simulink model "LinLongNormal_Aquila_ClawsGainSchedule_Discrete"  (R2017a)
settings: Solver=VariableStepAuto  StartTime=0.0  StopTime=50  RelTol=1e-3  EnableMultiTasking=on
PreLoadFcn:
  | AquilaDiscreteClawsParameters_GS
  | AquilaDiscreteModelParameters
model workspace: external: MAT-File (data not in the file)
undefined symbols (not defined in the file): AP_AltLoop_AltCmdLPFDenTau, AP_AltLoop_Kd0, AP_AltLoop_Ki0, AP_AltLoop_Ki_WindupMaxLim, AP_AltLoop_Ki_WindupMinLim, AP_AltLoop_Kp0, AP_ClimbRate_LPFDenTau, AP_ClimbRateLoop_ClimbRateCmdLPFDenTau, AP_ClimbRateLoop_Ki0, AP_ClimbRateLoop_Kp0, AP_ClimbRateLoop_LLFiltDenCoe0, AP_ClimbRateLoop_LLFiltNumCoe0, AP_ClimbRateLoop_MaxPitchCmdrad, AP_ClimbRateLoop_MinPitchCmdrad, AP_GndTrkLoop_CmdLPFDenTau, AP_GndTrkLoop_Kd0, AP_GndTrkLoop_Kp0, AP_GndTrkLoop_phiCmdMaxLimDeg, AP_GndTrkLoop_phiCmdMinLimDeg, AP_GndTrkLoop_phiRateCmdMaxLimDps, AP_GndTrkLoop_phiRateCmdMinLimDps, AP_PitchLoop_DerivLPFDenTau, AP_PitchLoop_Kd, AP_PitchLoop_Kff, AP_PitchLoop_Ki0, AP_PitchLoop_Kp0, AP_PitchLoop_Kq0, AP_PitchLoop_Notch1BWfactor, AP_PitchLoop_Notch1CosFreqNorm, AP_PitchLoop_qFdbkLFLLFiltDenCoe0, AP_PitchLoop_qFdbkLFLLFiltNumCoe0, AP_PitchLoop_qFdbkLLFiltDenCoe0, AP_PitchLoop_qFdbkLLFiltNumCoe0, AP_PitchLoop_thetaCmdLPFDenTau, AP_PitchLoop_wn_ElvRollOff, AP_PitchLoop_zeta_ElvRollOff, AP_PwrLoop_ClimbRateCmdLPFDenTau, AP_PwrLoop_Ki0, AP_PwrLoop_Kp0, AP_PwrLoop_Kvadv0, AP_PwrLoop_LLFiltDenCoe0, AP_PwrLoop_LLFiltNumCoe0, AP_PwrLoop_MaxThrCmdNorm, AP_PwrLoop_MinThrCmdNorm, AP_PwrLoop_wn_ThrRollOff, AP_PwrLoop_zeta_ThrRollOff, AP_RollLoop_ailCmdMaxLim, AP_RollLoop_ailCmdMinLim, AP_RollLoop_AilWindupMaxLim, AP_RollLoop_AilWindupMinLim, AP_RollLoop_Ki0, AP_RollLoop_Kp0, AP_RollLoop_KrollrateAdv0, AP_RollLoop_Notch1BWfactor, AP_RollLoop_Notch1CosFreqNorm, AP_RollLoop_pFdbkLFLLFiltDenCoe0, AP_RollLoop_pFdbkLFLLFiltNumCoe0, AP_RollLoop_pFdbkLLFiltDenCoe0, AP_RollLoop_pFdbkLLFiltNumCoe0, AP_RollLoop_phiErrLPFDenTau ... (+41)
libraries: discretizing x16, aerolibconvert2 x12, simulink x8
(part 1 of 2)
settings Model: Creator=The MathWorks, Inc.  LastModifiedBy=hbolandhemmat
settings DataIOCC: LimitDataPoints=on
settings OptimizationCC: LifeSpan=inf
settings DebuggingCC: AllowSymbolicDim=off  SFUnexpectedBacktrackingDiag=warning  SFNoUnconditionalDefaultTransitionDiag=warning  SFExecutionAtInitializationDiag=none
settings ModelReferenceCC: PropagateSignalLabelsOutOfModel=off
settings GRTTargetCC: TargetLangStandard=C89/C90 (ANSI)
settings ConfigComp: CovMetricSettings=dw  CovHtmlReporting=on  CovSaveCumulativeToWorkspaceVar=on  CovSaveSingleToWorkspaceVar=on  CovExternalEMLEnable=off

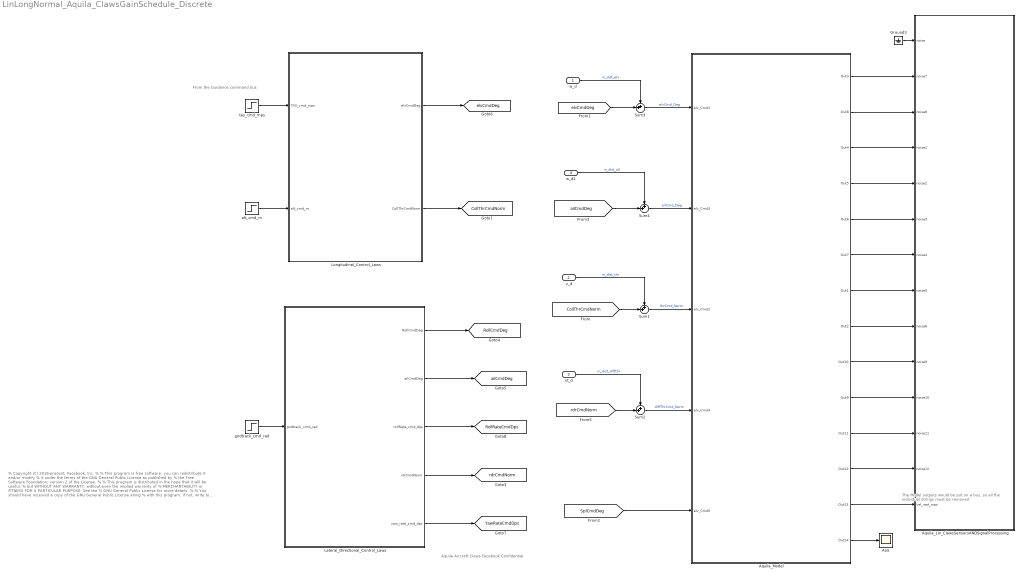
== system LinLongNormal_Aquila_ClawsGainSchedule_Discrete ==
  note: From the Guidance command bus
  note: Aquila Aircraft Claws
      | Facebook Confidential
  note: The Model outputs would be put on a bus, so all
      | the individual strings must be removed
  note: % Copyright (C) 2018-present, Facebook, Inc.
      | %
      | % This program is free software; you can redistribute it and/or modify
      | % it under the terms of the GNU General Public License as published by
      | % the Free Software Foundation; version 2 of the License.
      | %
      | % This program is distributed in the hope that it will be useful,
      | % but WITHOUT ANY WARRANTY; without even the implied warranty of
      | % MERCHANTABILITY or FITNESS FOR A PARTICULAR PURPOSE. See the
      | % GNU General Public License for more details.
      | %
      | % You should have received a copy of the GNU General Public License along
      | % with this program; if not, write to the Free Software Foundation, Inc.,
      | % 51 Franklin Street, Fifth Floor, Boston, MA 02110-1301 USA.
  w_d : Inport
  v_d : Inport  Port=2
  nt_d : Inport  Port=3
  w_d1 : Inport  Port=4
  AoS : Scope
  Aquila_Lin_ClawsSensorsANDSignalProcessing : Subsystem
  Aquila_Model : Subsystem
  Ground3 : Ground
  Lateral_Directional_Control_Laws : Subsystem
  Longitudinal_Control_Laws : Subsystem
  Sum{1..4} (4 alike) : Sum  Inputs=++|
  alt_cmd_m : Step  After=0  SampleTime=0
  gndtrack_cmd_rad : Step  SampleTime=0
  tas_cmd_mps : Step  After=0  SampleTime=0
  tag scope: CollThrCmdNorm=global, RollCmdDeg=global, RollRateCmdDps=global, YawRateCmdDps=global, ailCmdDeg=global, elvCmdDeg=global, rdrCmdNorm=global
  wires:
  alt_cmd_m/1 -> Longitudinal_Control_Laws/2(alt_cmd_m)
  Longitudinal_Control_Laws/1(elvCmdDeg) -> [elvCmdDeg]
  Longitudinal_Control_Laws/2(CollThrCmdNorm) -> [CollThrCmdNorm]
  w_d/1 -> Sum3/1  "in_dist_elv"
  Sum3/1 -> Aquila_Model/1(elv_Cmd1)  "elvCmd_Deg"
  Ground3/1 -> Aquila_Lin_ClawsSensorsANDSignalProcessing/1(noise)
  Aquila_Model/4(Out5) -> Aquila_Lin_ClawsSensorsANDSignalProcessing/5(noise2)
  Aquila_Model/3(Out4) -> Aquila_Lin_ClawsSensorsANDSignalProcessing/4(noise1)
  Aquila_Model/6(Out7) -> Aquila_Lin_ClawsSensorsANDSignalProcessing/7(noise4)
  Aquila_Model/1(Out3) -> Aquila_Lin_ClawsSensorsANDSignalProcessing/2(noise7)
  Aquila_Model/7(Out1) -> Aquila_Lin_ClawsSensorsANDSignalProcessing/8(noise5)
  Aquila_Model/8(Out2) -> Aquila_Lin_ClawsSensorsANDSignalProcessing/9(noise6)
  Aquila_Model/2(Out8) -> Aquila_Lin_ClawsSensorsANDSignalProcessing/3(noise8)
  v_d/1 -> Sum1/1  "in_dist_thr"
  Sum1/1 -> Aquila_Model/3(elv_Cmd2)  "thrCmd_Norm"
  Aquila_Model/5(Out6) -> Aquila_Lin_ClawsSensorsANDSignalProcessing/6(noise3)
  tas_cmd_mps/1 -> Longitudinal_Control_Laws/1(TAS_cmd_mps)
  [CollThrCmdNorm] -> Sum1/2
  [elvCmdDeg] -> Sum3/2
  Aquila_Model/9(Out10) -> Aquila_Lin_ClawsSensorsANDSignalProcessing/10(noise9)
  Aquila_Model/10(Out9) -> Aquila_Lin_ClawsSensorsANDSignalProcessing/11(noise10)
  Aquila_Model/11(Out11) -> Aquila_Lin_ClawsSensorsANDSignalProcessing/12(noise11)
  Aquila_Model/12(Out12) -> Aquila_Lin_ClawsSensorsANDSignalProcessing/13(noise12)
  Aquila_Model/13(Out13) -> Aquila_Lin_ClawsSensorsANDSignalProcessing/14(vel_ned_mps)
  Sum2/1 -> Aquila_Model/4(elv_Cmd4)  "diffThrCmd_Norm"
  [rdrCmdNorm] -> Sum2/2
  nt_d/1 -> Sum2/1  "in_dist_diffthr"
  Aquila_Model/14(Out14) -> AoS/1
  w_d1/1 -> Sum4/1  "in_dist_ail"
  [ailCmdDeg] -> Sum4/2
  Sum4/1 -> Aquila_Model/2(elv_Cmd3)  "ailCmd_Deg"
  [SplCmdDeg] -> Aquila_Model/5(elv_Cmd5)
  gndtrack_cmd_rad/1 -> Lateral_Directional_Control_Laws/1(gndtrack_cmd_rad)
  Lateral_Directional_Control_Laws/2(ailCmdDeg) -> [ailCmdDeg]
  Lateral_Directional_Control_Laws/1(RollCmdDeg) -> [RollCmdDeg]
  Lateral_Directional_Control_Laws/4(rdrCmdNorm) -> [rdrCmdNorm]
  Lateral_Directional_Control_Laws/5(yaw_rate_cmd_dps) -> [YawRateCmdDps]
  Lateral_Directional_Control_Laws/3(rollRate_cmd_dps) -> [RollRateCmdDps]

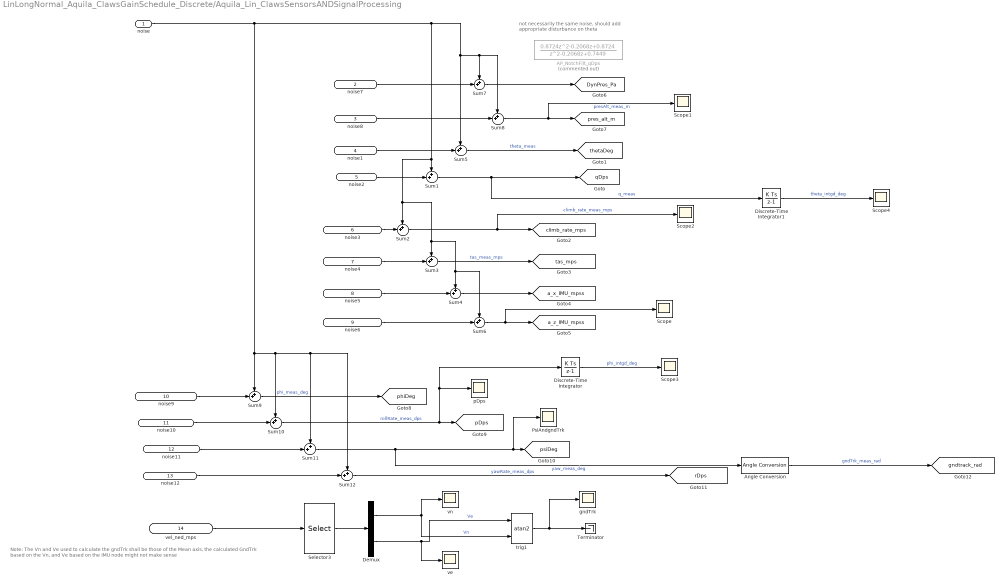
== system LinLongNormal_Aquila_ClawsGainSchedule_Discrete/Aquila_Lin_ClawsSensorsANDSignalProcessing ==
  note: Note: The Vn and Ve used to calculate the gndTrk shall be those of the Mean axis, the
      | calculated GndTrk based on the Vn, and Ve based on the IMU node might not make sense
  note: not necessarily the same noise,
      | should add appropriate disturbance on theta
  noise : Inport
  noise7 : Inport  Port=2
  noise8 : Inport  Port=3
  noise1 : Inport  Port=4
  noise2 : Inport  Port=5
  noise3 : Inport  Port=6
  noise4 : Inport  Port=7
  noise5 : Inport  Port=8
  noise6 : Inport  Port=9
  noise9 : Inport  Port=10
  noise10 : Inport  Port=11
  noise11 : Inport  Port=12
  noise12 : Inport  Port=13
  vel_ned_mps : Inport  Port=14
  AP_NotchFilt_qDps : DiscreteTransferFcn  Commented=on  Numerator=[0.8724 -0.2068 0.8724]  Denominator=[1 -0.2068 0.7449]  SampleTime=Ts
  Angle Conversion : aerolibconvert2/Angle Conversion  IU=deg  OU=rad
  Demux : Demux  Outputs=2
  Discrete-Time Integrator : DiscreteIntegrator  gainval=1  InitialConditionSetting=State (most efficient)  SampleTime=-1  ICPrevOutput=DiscIntNeverNeededParam  ICPrevScaledInput=DiscIntNeverNeededParam
  Discrete-Time Integrator1 : DiscreteIntegrator  gainval=1  InitialConditionSetting=State (most efficient)  SampleTime=-1  ICPrevOutput=DiscIntNeverNeededParam  ICPrevScaledInput=DiscIntNeverNeededParam
  PsiAndgndTrk : Scope
  Scope{,1..4} (5 alike) : Scope
  Selector3 : Selector  InputPortWidth=3  IndexOptions=Index vector (dialog)  Indices=1:2  OutputSizes=1
  Sum{1..12} (12 alike) : Sum  Inputs=++|
  Terminator : Terminator
  gndTrk : Scope
  pDps : Scope
  trig1 : Trigonometry  Operator=atan2
  ve : Scope
  vn : Scope
  tag scope: DynPres_Pa=global, a_x_IMU_mpss=global, a_z_IMU_mpss=global, climb_rate_mps=global, gndtrack_rad=global, pDps=global, phiDeg=global, pres_alt_m=global, psiDeg=global, qDps=global, rDps=global, tas_mps=global, thetaDeg=global
  wires:
  noise1/1 -> Sum5/2
  noise2/1 -> Sum1/2
  Sum5/1 -> [thetaDeg]  "theta_meas"
  Sum1/1 -> Discrete-Time Integrator1/1, [qDps]  "q_meas"
  noise3/1 -> Sum2/2
  Sum2/1 -> Scope2/1, [climb_rate_mps]  "climb_rate_meas_mps"
  noise4/1 -> Sum3/2
  Sum3/1 -> [tas_mps]  "tas_meas_mps"
  noise5/1 -> Sum4/2
  Sum4/1 -> [a_x_IMU_mpss]
  noise6/1 -> Sum6/2
  Sum6/1 -> Scope/1, [a_z_IMU_mpss]
  noise7/1 -> Sum7/2
  Sum7/1 -> [DynPres_Pa]
  noise8/1 -> Sum8/2
  Sum8/1 -> Scope1/1, [pres_alt_m]  "presAlt_meas_m"
  noise9/1 -> Sum9/2
  noise/1 -> Sum12/1, Sum11/1, Sum10/1, Sum9/1, Sum5/1, Sum8/1, Sum7/1, Sum6/1, Sum4/1, Sum3/1, Sum2/1, Sum1/1
  noise10/1 -> Sum10/2
  noise12/1 -> Sum12/2
  noise11/1 -> Sum11/2
  Sum9/1 -> [phiDeg]  "phi_meas_deg"
  Sum10/1 -> Discrete-Time Integrator/1, pDps/1, [pDps]  "rollRate_meas_dps"
  Sum11/1 -> PsiAndgndTrk/1, [psiDeg], Angle Conversion/1  "yaw_meas_deg"
  Sum12/1 -> [rDps]  "yawRate_meas_dps"
  Selector3/1 -> Demux/1
  Demux/2 -> trig1/1, ve/1  "Ve"
  Demux/1 -> vn/1, trig1/2  "Vn"
  vel_ned_mps/1 -> Selector3/1
  trig1/1 -> Terminator/1, gndTrk/1
  Angle Conversion/1 -> [gndtrack_rad]  "gndTrk_meas_rad"
  Discrete-Time Integrator/1 -> Scope3/1  "phi_intgd_deg"
  Discrete-Time Integrator1/1 -> Scope4/1  "theta_intgd_deg"

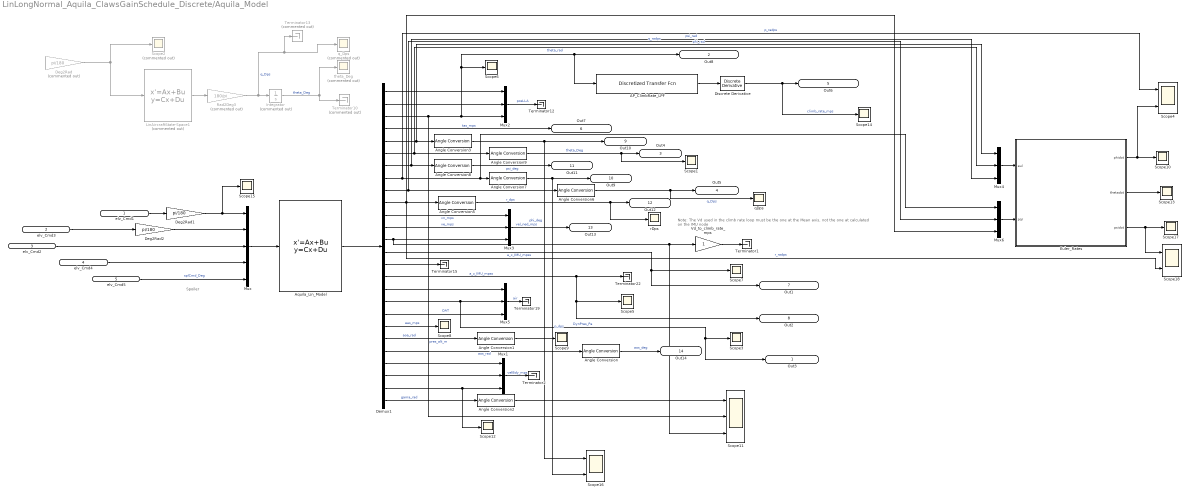
== system LinLongNormal_Aquila_ClawsGainSchedule_Discrete/Aquila_Model ==
  note: Spoiler
  note: Note: The Vd used in the climb rate loop must be the one at the Mean axis,
      | not the one at calculated on the IMU node
  elv_Cmd1 : Inport
  elv_Cmd3 : Inport  Port=2
  elv_Cmd2 : Inport  Port=3
  elv_Cmd4 : Inport  Port=4
  elv_Cmd5 : Inport  Port=5
  AP_ClimbRate_LPF : discretizing/Discretized Transfer Fcn  Numerator=[1]  Denominator=[AP_ClimbRate_LPFDenTau 1]  AbsTol=auto  SampleTime=Ts  method=zoh  Wc=1
  Angle Conversion{,1..3,5..9} (9 alike) : aerolibconvert2/Angle Conversion  IU=rad  OU=deg
  Aquila_Lin_Model : StateSpace  A=LIN_AC_S_A  B=LIN_AC_S_B  C=LIN_AC_S_C  D=LIN_AC_S_D  X0=0
  Deg2Rad : Gain  Commented=on  Gain=pi/180
  Deg2Rad1 : Gain  Gain=pi/180
  Deg2Rad2 : Gain  Gain=pi/180
  Demux1 : Demux  Outputs=26
  Discrete Derivative : simulink/Discrete/Discrete Derivative  gainval=1.0  ICPrevScaledInput=0.0  OutMin=[]  OutMax=[]  OutDataType=fixdt(1, 16)  OutScaling=2^-10  DoSatur=off
  Euler_Rates : Subsystem
  Integrator : Integrator  Commented=on
  LinAircraftState-Space1 : StateSpace  Commented=on  A=LIN_AC_S_A  B=LIN_AC_S_B  C=LIN_AC_S_C  D=LIN_AC_S_D  X0=0
  Mux : Mux  Inputs=5
  Mux{1..6} (6 alike) : Mux  Inputs=3
  Rad2Deg3 : Gain  Commented=on  Gain=180/pi
  Scope{1,3,5..10,12..15,17} (13 alike) : Scope
  Scope11 : Scope  NumInputPorts=3
  Scope16 : Scope  NumInputPorts=2
  Scope18 : Scope  NumInputPorts=2
  Scope2 : Scope  Commented=on
  Scope4 : Scope  NumInputPorts=2
  Terminator{1..2,12,15,19,22} (6 alike) : Terminator
  Terminator10 : Terminator  Commented=on
  Terminator13 : Terminator  Commented=on
  Vd_to_climb_rate_mps : Gain
  qDps : Scope
  q_Dps : Scope  Commented=on
  rDps : Scope
  theta_Deg : Scope  Commented=on
  Out3 : Outport
  Out8 : Outport  Port=2
  Out4 : Outport  Port=3
  Out5 : Outport  Port=4
  Out6 : Outport  Port=5
  Out7 : Outport  Port=6
  Out1 : Outport  Port=7
  Out2 : Outport  Port=8
  Out10 : Outport  Port=9
  Out9 : Outport  Port=10
  Out11 : Outport  Port=11
  Out12 : Outport  Port=12
  Out13 : Outport  Port=13
  Out14 : Outport  Port=14
  wires:
  LinAircraftState-Space1/1 -> Rad2Deg3/1
  Deg2Rad/1 -> LinAircraftState-Space1/1, Scope2/1
  Integrator/1 -> Terminator10/1, theta_Deg/1  "theta_Deg"
  Rad2Deg3/1 -> q_Dps/1, Terminator13/1, Integrator/1  "q_Dps"
  elv_Cmd5/1 -> Mux/5  "splCmd_Deg"
  Mux/1 -> Aquila_Lin_Model/1
  Deg2Rad1/1 -> Scope15/1, Mux/1
  elv_Cmd1/1 -> Deg2Rad1/1
  Demux1/8 -> Scope4/1, Mux6/1, Angle Conversion7/1  "p_radps"
  Demux1/15 -> Terminator15/1
  Demux1/3 -> Scope6/1, AP_ClimbRate_LPF/1, Out8/1, Mux2/3, Scope11/2  "pres_alt_m"
  Mux2/1 -> Terminator12/1  "posLLA"
  Demux1/2 -> Mux2/2
  Demux1/18 -> Out3/1, Scope3/1, Mux5/2  "DynPres_Pa"
  Demux1/17 -> Mux5/1
  Demux1/1 -> Mux2/1
  Demux1/19 -> Mux5/3  "OAT"
  Mux5/1 -> Terminator19/1  "air"
  Demux1/5 -> Mux4/1, Angle Conversion3/1  "phi_rad"
  Demux1/14 -> Out1/1, Scope7/1  "a_x_IMU_mpss"
  Demux1/16 -> Out2/1, Scope5/1, Terminator22/1  "a_z_IMU_mpss"
  Demux1/7 -> Mux4/3, Angle Conversion8/1  "psi_rad"
  Demux1/6 -> Mux4/2, Angle Conversion9/1  "theta_rad"
  Angle Conversion9/1 -> Scope1/1, Out4/1  "theta_Deg"
  Demux1/9 -> Mux6/2, Angle Conversion6/1  "q_radps"
  Angle Conversion6/1 -> qDps/1, Out5/1  "q_Dps"
  Aquila_Lin_Model/1 -> Demux1/1
  Demux1/4 -> Out7/1  "tas_mps"
  Vd_to_climb_rate_mps/1 -> Terminator1/1
  Demux1/20 -> Scope8/1  "eas_mps"
  Demux1/21 -> Angle Conversion1/1  "aoa_rad"
  Demux1/22 -> Angle Conversion/1  "aos_rad"
  Demux1/23 -> Mux1/1
  Demux1/24 -> Mux1/2
  Demux1/26 -> Angle Conversion2/1  "gama_rad"
  Angle Conversion/1 -> Out14/1  "aos_deg"
  Angle Conversion1/1 -> Scope9/1
  Angle Conversion2/1 -> Scope11/1
  elv_Cmd4/1 -> Mux/4
  AP_ClimbRate_LPF/1 -> Discrete Derivative/1
  Discrete Derivative/1 -> Scope14/1, Out6/1  "climb_rate_mps"
  Demux1/10 -> Scope18/2, Mux6/3, Angle Conversion5/1  "r_radps"
  Angle Conversion5/1 -> rDps/1, Out12/1  "r_dps"
  Angle Conversion7/1 -> Scope16/2, Out9/1  "p_dps"
  Angle Conversion3/1 -> Scope16/1, Out10/1  "phi_deg"
  Angle Conversion8/1 -> Out11/1  "psi_deg"
  elv_Cmd2/1 -> Mux/3
  elv_Cmd3/1 -> Deg2Rad2/1
  Mux1/1 -> Terminator2/1  "velBdy_mps"
  Demux1/25 -> Scope12/1, Mux1/3
  Demux1/11 -> Mux3/1  "vn_mps"
  Demux1/12 -> Mux3/2  "ve_mps"
  Demux1/13 -> Scope11/3, Vd_to_climb_rate_mps/1, Mux3/3
  Mux3/1 -> Out13/1  "vel_ned_mps"
  Mux4/1 -> Euler_Rates/1(eul)
  Mux6/1 -> Euler_Rates/2(pqr)
  Euler_Rates/1(phidot) -> Scope4/2, Scope10/1
  Euler_Rates/2(thetadot) -> Scope13/1
  Euler_Rates/3(psidot) -> Scope18/1, Scope17/1
  Deg2Rad2/1 -> Mux/2

== system LinLongNormal_Aquila_ClawsGainSchedule_Discrete/Lateral_Directional_Control_Laws ==
  note: Aquila Aircraft Claws
      | Facebook Confidential
  gndtrack_cmd_rad : Inport
  GndTrkLoop : Subsystem
  RollLoop : Subsystem
  YawLoop : Subsystem
  RollCmdDeg : Outport
  ailCmdDeg : Outport  Port=2
  rollRate_cmd_dps : Outport  Port=3
  rdrCmdNorm : Outport  Port=4
  yaw_rate_cmd_dps : Outport  Port=5
  wires:
  gndtrack_cmd_rad/1 -> GndTrkLoop/1(alt_cmd_m)
  RollLoop/1(ail_cmd_RollRateLoop_deg) -> ailCmdDeg/1
  YawLoop/1(Rdr_cmd_YawRateLoop_norm) -> rdrCmdNorm/1
  YawLoop/2(yaw_rate_cmd_dps) -> yaw_rate_cmd_dps/1
  GndTrkLoop/1(Phi_cmd_deg) -> RollCmdDeg/1, RollLoop/1(phi_cmd_deg)
  RollLoop/3(phi_err_filt) -> YawLoop/1(alt_cmd_m)
  RollLoop/2(PhiRateCmd_Dps) -> rollRate_cmd_dps/1
  GndTrkLoop/2(PhiRate_cmd_dps) -> RollLoop/2(phiRateCmd_Dps)

== system LinLongNormal_Aquila_ClawsGainSchedule_Discrete/Longitudinal_Control_Laws ==
  note: The ClimbRate loop might be replaced by the Nz loop
      | in the future depending on the overall loop performance
      | and availability of the Nz signal in terms of SNR
  note: Aquila Aircraft Longitudinal Claws
      | Facebook Confidential
  TAS_cmd_mps : Inport
  alt_cmd_m : Inport  Port=2
  AltitudeLoop : Subsystem
  ClimbRateLoop : Subsystem
  PitchLoop : Subsystem
  PwrLoop : Subsystem
  SpeedLoop : Subsystem
  elvCmdDeg : Outport
  CollThrCmdNorm : Outport  Port=2
  wires:
  PitchLoop/1(elv_Cmd_PitchLoop) -> elvCmdDeg/1  "elvCmdDeg_PitchLoop"
  PwrLoop/1(CollThr_Cmd_PwrLoop) -> CollThrCmdNorm/1
  alt_cmd_m/1 -> AltitudeLoop/1(alt_cmd_m)
  [climb_rate_mps] -> PwrLoop/2(climb_rate_mps)
  [climb_rate_mps] -> ClimbRateLoop/3(climb_rate_mps)
  [pres_alt_m] -> AltitudeLoop/2(alt_m)
  SpeedLoop/1(climb_rate_cmd_spdloop) -> ClimbRateLoop/1(climb_rate_cmd_spdloop)
  ClimbRateLoop/1(theta_Cmd) -> PitchLoop/1(theta_Cmd)
  [tas_mps] -> PwrLoop/3(TAS_mps)
  AltitudeLoop/1(climb_rate_cmd_altloop_mps) -> PwrLoop/1(climb_rate_altloop_cmd_mps), ClimbRateLoop/2(climb_rate_cmd_altloop_mps)
  [climb_rate_mps] -> AltitudeLoop/3(climb_rate_mps)
  TAS_cmd_mps/1 -> SpeedLoop/1(TAS_cmd_mps)
  [tas_mps] -> SpeedLoop/2(TAS_mps)

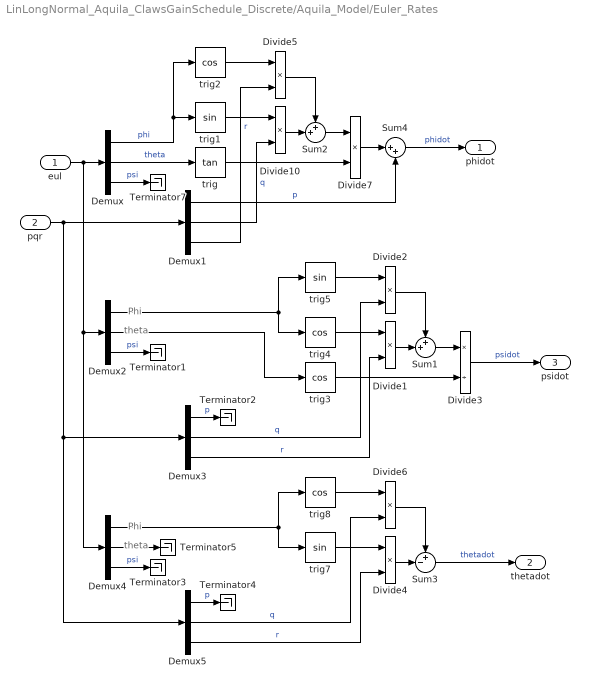
== system LinLongNormal_Aquila_ClawsGainSchedule_Discrete/Aquila_Model/Euler_Rates ==
  note: theta
  note: Phi
  note: theta
  note: Phi
  eul : Inport
  pqr : Inport  Port=2
  Demux{,1..5} (6 alike) : Demux  Outputs=3
  Divide{1..2,4..7,10} (7 alike) : Product  Inputs=**
  Divide3 : Product  Inputs=*/
  Sum1 : Sum  Inputs=++|
  Sum2 : Sum  Inputs=++|
  Sum3 : Sum  Inputs=+-|
  Sum4 : Sum  Inputs=|++
  Terminator{1..5,7} (6 alike) : Terminator
  trig : Trigonometry  Operator=tan
  trig1 : Trigonometry
  trig{2..4,8} (4 alike) : Trigonometry  Operator=cos
  trig5 : Trigonometry
  trig7 : Trigonometry
  phidot : Outport
  thetadot : Outport  Port=2
  psidot : Outport  Port=3
  wires:
  Divide5/1 -> Sum2/1
  trig2/1 -> Divide5/1
  Divide7/1 -> Sum4/1
  Demux1/1 -> Sum4/2  "p"
  trig1/1 -> Divide10/1
  Demux1/3 -> Divide5/2  "r"
  Demux1/2 -> Divide10/2  "q"
  Sum2/1 -> Divide7/1
  trig/1 -> Divide7/2
  Sum4/1 -> phidot/1  "phidot"
  Divide10/1 -> Sum2/2
  Demux/3 -> Terminator7/1  "psi"
  Divide2/1 -> Sum1/1
  trig5/1 -> Divide2/1
  trig4/1 -> Divide1/1
  Demux/1 -> trig2/1, trig1/1  "phi"
  Demux/2 -> trig/1  "theta"
  Sum1/1 -> Divide3/1
  trig3/1 -> Divide3/2
  Divide3/1 -> psidot/1  "psidot"
  Divide1/1 -> Sum1/2
  Demux3/2 -> Divide2/2  "q"
  Demux3/3 -> Divide1/2  "r"
  Demux2/1 -> trig5/1, trig4/1
  Demux2/2 -> trig3/1
  Demux2/3 -> Terminator1/1  "psi"
  Demux3/1 -> Terminator2/1  "p"
  pqr/1 -> Demux1/1, Demux3/1, Demux5/1
  Divide6/1 -> Sum3/1
  trig8/1 -> Divide6/1
  trig7/1 -> Divide4/1
  Sum3/1 -> thetadot/1  "thetadot"
  Divide4/1 -> Sum3/2
  Demux5/2 -> Divide6/2  "q"
  Demux5/3 -> Divide4/2  "r"
  eul/1 -> Demux2/1, Demux4/1, Demux/1
  Demux4/1 -> trig8/1, trig7/1
  Demux4/3 -> Terminator3/1  "psi"
  Demux5/1 -> Terminator4/1  "p"
  Demux4/2 -> Terminator5/1

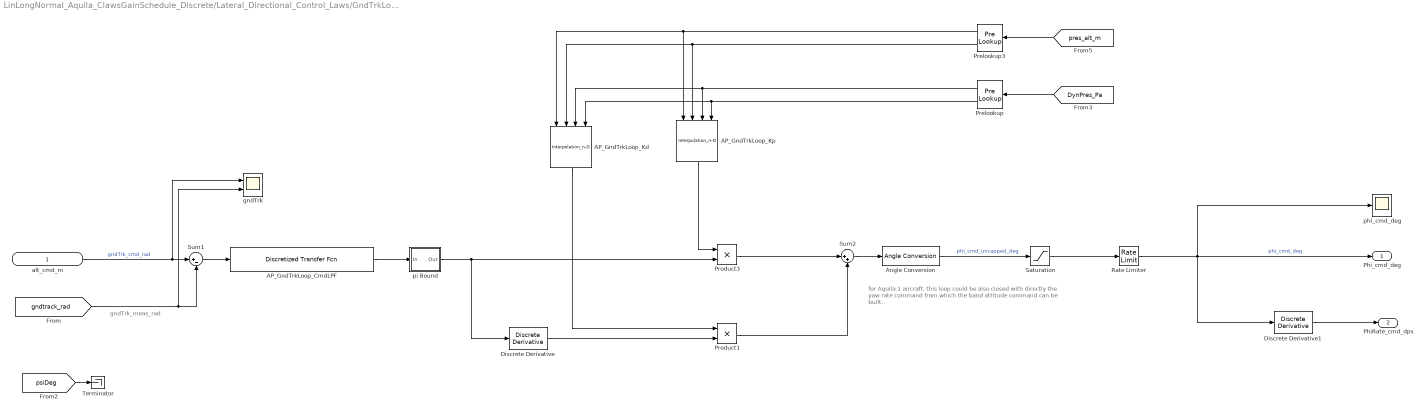
== system LinLongNormal_Aquila_ClawsGainSchedule_Discrete/Lateral_Directional_Control_Laws/GndTrkLoop ==
  note: gndTrk_meas_rad
  note: for Aquila 1 aircraft, this loop could be also closed with
      | directly the yaw rate command from which the band attitude
      | command can be built.
  alt_cmd_m : Inport
  AP_GndTrkLoop_CmdLPF : discretizing/Discretized Transfer Fcn  Numerator=[1]  Denominator=[AP_GndTrkLoop_CmdLPFDenTau 1]  AbsTol=auto  SampleTime=Ts  method=zoh  Wc=1
  AP_GndTrkLoop_Kd : Interpolation_n-D  Table=AP_GndTrkLoop_Kd0  ExtrapMethod=Clip  InternalRulePriority=Speed
  AP_GndTrkLoop_Kp : Interpolation_n-D  Table=AP_GndTrkLoop_Kp0  ExtrapMethod=Clip  InternalRulePriority=Speed
  Angle Conversion : aerolibconvert2/Angle Conversion  IU=rad  OU=deg
  Discrete Derivative : simulink/Discrete/Discrete Derivative  gainval=1.0  ICPrevScaledInput=0.0  OutMin=[]  OutMax=[]  OutDataType=fixdt(1, 16)  OutScaling=2^-10  DoSatur=off
  Discrete Derivative1 : simulink/Discrete/Discrete Derivative  gainval=1.0  ICPrevScaledInput=0.0  OutMin=[]  OutMax=[]  OutDataType=fixdt(1, 16)  OutScaling=2^-10  DoSatur=off
  Prelookup : PreLookup  BreakpointsData=45:15:150  ExtrapMethod=Linear
  Prelookup3 : PreLookup  BreakpointsData=0:1500:12000  ExtrapMethod=Linear
  Product1 : Product
  Product3 : Product
  Rate Limiter : RateLimiter  RisingSlewLimit=AP_GndTrkLoop_phiRateCmdMaxLimDps  FallingSlewLimit=AP_GndTrkLoop_phiRateCmdMinLimDps  SampleTimeMode=inherited
  Saturation : Saturate  UpperLimit=AP_GndTrkLoop_phiCmdMaxLimDeg  LowerLimit=AP_GndTrkLoop_phiCmdMinLimDeg
  Sum1 : Sum  Inputs=|+-
  Sum2 : Sum  Inputs=|++
  Terminator : Terminator
  gndTrk : Scope  NumInputPorts=2
  phi_cmd_deg : Scope
  pi Bound : Subsystem  mask(pi bound){}
      mask help: Bounds the input angle to [-pi, pi]. When -pi bound is exceeded the output wraps back to pi; when the pi bound is exceeded the output wraps back to -pi.
      mask Help:
      | Bounds the input angle to [-pi, pi]. When -pi bound is exceeded the output wraps back to pi; when the pi bound is exceeded the output wraps back to -pi.
      | <P><B>Input:</B> any angle in radians, from -Inf to Inf;</P>
      | <P><B>Output:</B> an angle in radians between -pi and pi.</P>
  Phi_cmd_deg : Outport
  PhiRate_cmd_dps : Outport  Port=2
  wires:
  alt_cmd_m/1 -> gndTrk/1, Sum1/1  "gndTrk_cmd_rad"
  [psiDeg] -> Terminator/1
  Product3/1 -> Sum2/1
  Sum1/1 -> AP_GndTrkLoop_CmdLPF/1
  Product1/1 -> Sum2/2
  Discrete Derivative/1 -> Product1/2
  Angle Conversion/1 -> Saturation/1  "phi_cmd_uncapped_deg"
  Sum2/1 -> Angle Conversion/1
  [gndtrack_rad] -> Sum1/2, gndTrk/2
  AP_GndTrkLoop_CmdLPF/1 -> pi Bound/1(In)
  pi Bound/1(Out) -> Product3/2, Discrete Derivative/1
  Discrete Derivative1/1 -> PhiRate_cmd_dps/1
  Saturation/1 -> Rate Limiter/1
  Rate Limiter/1 -> Discrete Derivative1/1, phi_cmd_deg/1, Phi_cmd_deg/1  "phi_cmd_deg"
  [DynPres_Pa] -> Prelookup/1
  Prelookup/2 -> AP_GndTrkLoop_Kd/4, AP_GndTrkLoop_Kp/4
  Prelookup/1 -> AP_GndTrkLoop_Kd/3, AP_GndTrkLoop_Kp/3
  [pres_alt_m] -> Prelookup3/1
  Prelookup3/1 -> AP_GndTrkLoop_Kd/1, AP_GndTrkLoop_Kp/1
  Prelookup3/2 -> AP_GndTrkLoop_Kd/2, AP_GndTrkLoop_Kp/2
  AP_GndTrkLoop_Kp/1 -> Product3/1
  AP_GndTrkLoop_Kd/1 -> Product1/1

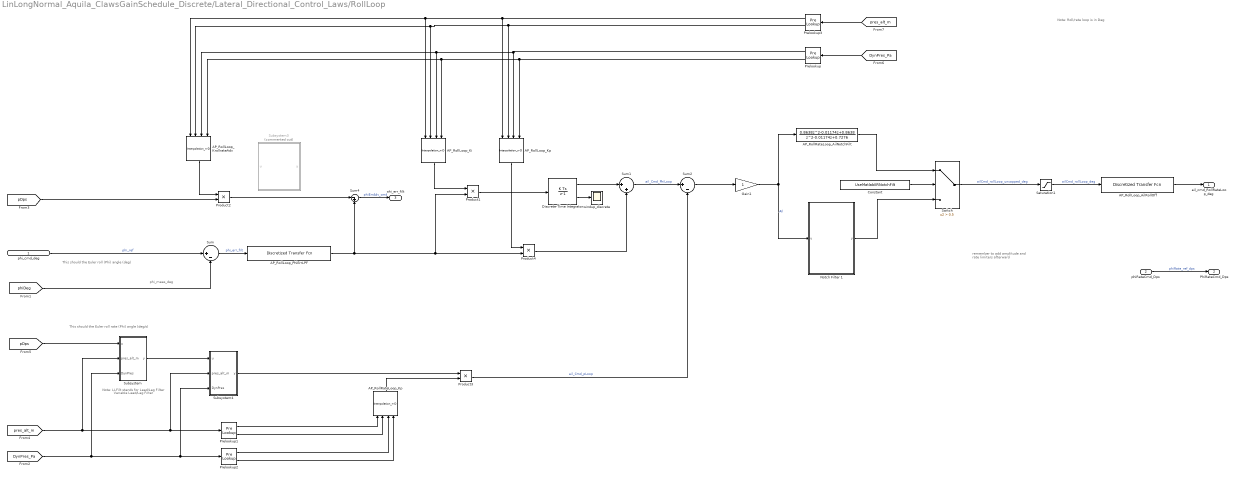
== system LinLongNormal_Aquila_ClawsGainSchedule_Discrete/Lateral_Directional_Control_Laws/RollLoop ==
  note: phi_meas_deg
  note: This should the Euler roll (Phi) angle (deg)
  note: This should the Euler roll rate (Phi) angle (deg/s)
  note: remember to add amplitude and
      | rate limiters afterward
  note: Note: Roll/rate loop is in Deg
  note: Variable Lead/Lag Filter
  note: Note: LLFilt stands for Lead/Lag Filter
  phi_cmd_deg : Inport
  phiRateCmd_Dps : Inport  Port=2
  AP_RollLoop_AilRollOff : discretizing/Discretized Transfer Fcn  Numerator=[AP_RollLoop_wn_AilRollOff^2]  Denominator=[1 2*AP_RollLoop_zeta_AilRollOff*AP_RollLoop_wn_AilRollOff AP_RollLoop_wn_AilRollOff^2]  AbsTol=auto  SampleTime=Ts  method=zoh  Wc=1
  AP_RollLoop_Ki : Interpolation_n-D  Table=AP_RollLoop_Ki0  ExtrapMethod=Clip  InternalRulePriority=Speed
  AP_RollLoop_Kp : Interpolation_n-D  Table=AP_RollLoop_Kp0  ExtrapMethod=Clip  InternalRulePriority=Speed
  AP_RollLoop_KrollrateAdv : Interpolation_n-D  Table=AP_RollLoop_KrollrateAdv0  ExtrapMethod=Clip  InternalRulePriority=Speed
  AP_RollLoop_PhiErrLPF : discretizing/Discretized Transfer Fcn  Numerator=[1]  Denominator=[AP_RollLoop_phiErrLPFDenTau 1]  AbsTol=auto  SampleTime=Ts  method=zoh  Wc=1
  AP_RollRateLoop_AilNotchFilt : DiscreteTransferFcn  Numerator=[0.8638 -0.01174 0.8638]  Denominator=[1 -0.01174 0.7276]  SampleTime=Ts
  AP_RollRateLoop_Kp : Interpolation_n-D  Table=AP_RollRateLoop_Kp0  InternalRulePriority=Speed
  Constant : Constant  Value=UseMatlabIIRNotchFilt
  Discrete-Time Integrator : DiscreteIntegrator  InitialConditionSetting=State (most efficient)  SampleTime=Ts  LimitOutput=on  UpperSaturationLimit=AP_RollLoop_AilWindupMaxLim  LowerSaturationLimit=AP_RollLoop_AilWindupMinLim  ShowSaturationPort=on  ICPrevOutput=DiscIntNeverNeededParam  ICPrevScaledInput=DiscIntNeverNeededParam
  Gain1 : Gain
  Notch Filter 1 : Subsystem
  Prelookup : PreLookup  BreakpointsData=45:15:150  ExtrapMethod=Linear
  Prelookup1 : PreLookup  BreakpointsData=0:1500:12000  ExtrapMethod=Linear
  Prelookup2 : PreLookup  BreakpointsData=45:15:150  ExtrapMethod=Linear
  Prelookup3 : PreLookup  BreakpointsData=0:1500:12000  ExtrapMethod=Linear
  Product{1..4} (4 alike) : Product
  Saturation1 : Saturate  UpperLimit=AP_RollLoop_ailCmdMaxLim  LowerLimit=AP_RollLoop_ailCmdMinLim
  Subsystem : Subsystem
  Subsystem3 : Subsystem  Commented=on
  Subsystem4 : Subsystem
  Sum : Sum  Inputs=|+-
  Sum1 : Sum  Inputs=|++
  Sum2 : Sum  Inputs=|+-
  Sum4 : Sum  Inputs=|-+
  Switch : Switch  Criteria=u2 > Threshold  Threshold=0.5
  windup_discrete : Scope
  ail_cmd_RollRateLoop_deg : Outport
  PhiRateCmd_Dps : Outport  Port=2
  phi_err_filt : Outport  Port=3
  wires:
  Product1/1 -> Discrete-Time Integrator/1
  phi_cmd_deg/1 -> Sum/1  "phi_ref"
  Product4/1 -> Sum1/2
  Discrete-Time Integrator/2 -> windup_discrete/1
  Discrete-Time Integrator/1 -> Sum1/1
  Switch/1 -> Saturation1/1  "ailCmd_rollLoop_uncapped_deg"
  Saturation1/1 -> AP_RollLoop_AilRollOff/1  "ailCmd_rollLoop_deg"
  [pDps] -> Product2/2
  phiRateCmd_Dps/1 -> PhiRateCmd_Dps/1  "phiRate_ref_dps"
  Sum1/1 -> Sum2/1  "ail_Cmd_PhiLoop"
  Sum2/1 -> Gain1/1
  Sum4/1 -> phi_err_filt/1  "phiErrAdv_cmd"
  [phiDeg] -> Sum/2
  Sum/1 -> AP_RollLoop_PhiErrLPF/1  "phi_err_filt"
  Product2/1 -> Sum4/1
  AP_RollLoop_PhiErrLPF/1 -> Sum4/2, Product1/2, Product4/2
  AP_RollRateLoop_AilNotchFilt/1 -> Switch/1
  Notch Filter 1/1(y) -> Switch/3
  Constant/1 -> Switch/2
  Gain1/1 -> Notch Filter 1/1(u), AP_RollRateLoop_AilNotchFilt/1  "Ail"
  AP_RollLoop_AilRollOff/1 -> ail_cmd_RollRateLoop_deg/1
  [DynPres_Pa] -> Subsystem4/3(DynPres), Prelookup2/1, Subsystem/3(DynPres)
  AP_RollRateLoop_Kp/1 -> Product3/2
  [pres_alt_m] -> Subsystem4/2(pres_alt_m), Prelookup1/1, Subsystem/2(pres_alt_m)
  Prelookup1/1 -> AP_RollRateLoop_Kp/1
  Prelookup1/2 -> AP_RollRateLoop_Kp/2
  Prelookup2/1 -> AP_RollRateLoop_Kp/3
  Prelookup2/2 -> AP_RollRateLoop_Kp/4
  Subsystem4/1(y) -> Product3/1
  [pDps] -> Subsystem/1(u)
  Subsystem/1(y) -> Subsystem4/1(u)
  Product3/1 -> Sum2/2  "ail_Cmd_pLoop"
  [DynPres_Pa] -> Prelookup/1
  Prelookup/2 -> AP_RollLoop_Kp/4, AP_RollLoop_KrollrateAdv/4, AP_RollLoop_Ki/4
  Prelookup/1 -> AP_RollLoop_Kp/3, AP_RollLoop_KrollrateAdv/3, AP_RollLoop_Ki/3
  [pres_alt_m] -> Prelookup3/1
  Prelookup3/2 -> AP_RollLoop_KrollrateAdv/2, AP_RollLoop_Ki/2, AP_RollLoop_Kp/2
  AP_RollLoop_Ki/1 -> Product1/1
  Prelookup3/1 -> AP_RollLoop_KrollrateAdv/1, AP_RollLoop_Ki/1, AP_RollLoop_Kp/1
  AP_RollLoop_KrollrateAdv/1 -> Product2/1
  AP_RollLoop_Kp/1 -> Product4/1

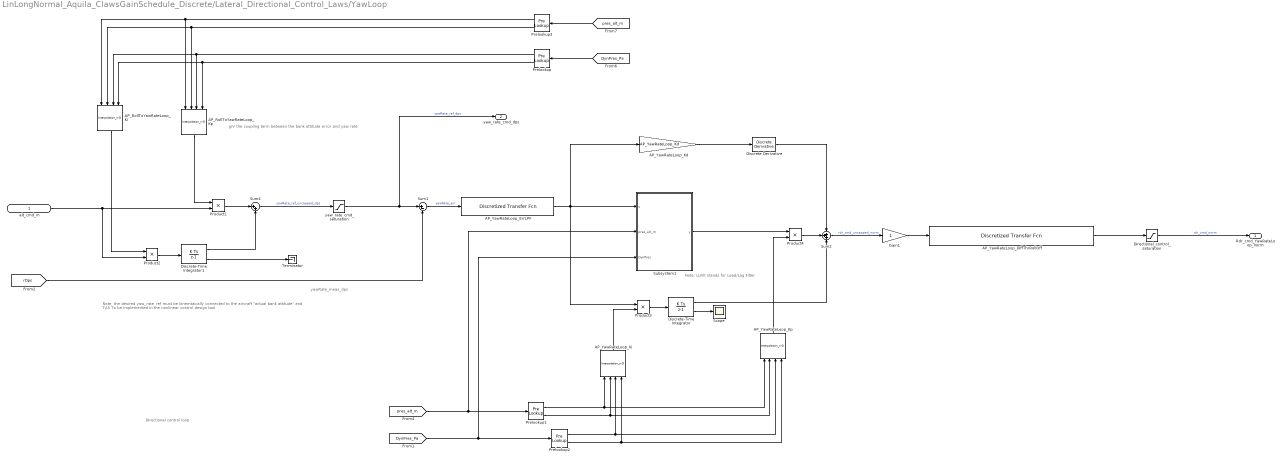
== system LinLongNormal_Aquila_ClawsGainSchedule_Discrete/Lateral_Directional_Control_Laws/YawLoop ==
  note: yawRate_meas_dps
  note: g/V the coupling term between the bank attitude error and yaw rate
  note: Directional control loop
  note: Note, the desired yaw_rate_ref must be kinemtaically connected to the aircraft "actual bank attitude" and TAS
      | To be implemented in the nonlinear control design tool
  note: Note: LLFilt stands for Lead/Lag Filter
  alt_cmd_m : Inport
  AP_RollToYawRateLoop_Ki : Interpolation_n-D  Table=AP_RollToYawRateLoop_Ki0  ExtrapMethod=Clip  InternalRulePriority=Speed
  AP_RollToYawRateLoop_Kp : Interpolation_n-D  Table=AP_RollToYawRateLoop_Kp0  ExtrapMethod=Clip  InternalRulePriority=Speed
  AP_YawRateLoop_DiffThrRollOff : discretizing/Discretized Transfer Fcn  Numerator=[AP_YawRateLoop_wn_DiffThrRollOff^2]  Denominator=[1 2*AP_YawRateLoop_zeta_DiffThrRollOff*AP_YawRateLoop_wn_DiffThrRollOff AP_YawRateLoop_wn_DiffThrRollOff^2]  AbsTol=auto  SampleTime=Ts  method=zoh  Wc=1
  AP_YawRateLoop_ErrLPF : discretizing/Discretized Transfer Fcn  Numerator=[1]  Denominator=[AP_YawRateLoop_ErrLPFDenTau 1]  AbsTol=auto  SampleTime=Ts  method=zoh  Wc=1
  AP_YawRateLoop_Kd : Gain  Gain=AP_YawRateLoop_Kd
  AP_YawRateLoop_Ki : Interpolation_n-D  Table=AP_YawRateLoop_Ki0  ExtrapMethod=Clip  InternalRulePriority=Speed
  AP_YawRateLoop_Kp : Interpolation_n-D  Table=AP_YawRateLoop_Kp0  ExtrapMethod=Clip  InternalRulePriority=Speed
  Directional_control_saturation : Saturate  UpperLimit=AP_YawRateLoop_RdrCmdMaxLimNorm  LowerLimit=AP_YawRateLoop_RdrCmdMinLimNorm
  Discrete Derivative : simulink/Discrete/Discrete Derivative  gainval=1.0  ICPrevScaledInput=0.0  OutMin=[]  OutMax=[]  OutDataType=fixdt(1, 16)  OutScaling=2^-10  DoSatur=off
  Discrete-Time Integrator : DiscreteIntegrator  InitialConditionSetting=State (most efficient)  SampleTime=Ts  LimitOutput=on  UpperSaturationLimit=AP_YawRateLoop_RdrWindupMaxLim  LowerSaturationLimit=AP_YawRateLoop_RdrWindupMinLim  ShowSaturationPort=on  ICPrevOutput=DiscIntNeverNeededParam  ICPrevScaledInput=DiscIntNeverNeededParam
  Discrete-Time Integrator1 : DiscreteIntegrator  InitialConditionSetting=State (most efficient)  SampleTime=Ts  LimitOutput=on  UpperSaturationLimit=AP_RollToYawRateLoop_YawRateWindupMaxLim  LowerSaturationLimit=AP_RollToYawRateLoop_YawRateWindupMinLim  ShowSaturationPort=on  ICPrevOutput=DiscIntNeverNeededParam  ICPrevScaledInput=DiscIntNeverNeededParam
  Gain1 : Gain
  Prelookup : PreLookup  BreakpointsData=45:15:150  ExtrapMethod=Linear
  Prelookup1 : PreLookup  BreakpointsData=0:1500:12000  ExtrapMethod=Linear
  Prelookup2 : PreLookup  BreakpointsData=45:15:150  ExtrapMethod=Linear
  Prelookup3 : PreLookup  BreakpointsData=0:1500:12000  ExtrapMethod=Linear
  Product{1..4} (4 alike) : Product
  Scope : Scope
  Subsystem1 : Subsystem
  Sum1 : Sum  Inputs=|+-
  Sum2 : Sum  Inputs=+++
  Sum4 : Sum  Inputs=|++
  Terminator : Terminator
  yaw_rate_cmd_saturation : Saturate  UpperLimit=AP_YawRateLoop_YawRateMaxLimDps  LowerLimit=AP_YawRateLoop_YawRateMinLimDps
  Rdr_cmd_YawRateLoop_norm : Outport
  yaw_rate_cmd_dps : Outport  Port=2
  wires:
  Product4/1 -> Sum2/2
  Product3/1 -> Discrete-Time Integrator/1
  Directional_control_saturation/1 -> Rdr_cmd_YawRateLoop_norm/1  "rdr_cmd_norm"
  Sum1/1 -> AP_YawRateLoop_ErrLPF/1  "yawRate_err"
  [rDps] -> Sum1/2
  Sum2/1 -> Gain1/1  "rdr_cmd_uncapped_norm"
  Discrete-Time Integrator/2 -> Scope/1
  AP_YawRateLoop_Kd/1 -> Discrete Derivative/1
  Discrete-Time Integrator/1 -> Sum2/3
  Discrete Derivative/1 -> Sum2/1
  Gain1/1 -> AP_YawRateLoop_DiffThrRollOff/1
  alt_cmd_m/1 -> Product2/2, Product1/2
  Product2/1 -> Discrete-Time Integrator1/1
  Sum4/1 -> yaw_rate_cmd_saturation/1  "yawRate_ref_uncapped_dps"
  Discrete-Time Integrator1/2 -> Terminator/1
  AP_YawRateLoop_DiffThrRollOff/1 -> Directional_control_saturation/1
  Discrete-Time Integrator1/1 -> Sum4/2
  Product1/1 -> Sum4/1
  yaw_rate_cmd_saturation/1 -> yaw_rate_cmd_dps/1, Sum1/1  "yawRate_ref_dps"
  [DynPres_Pa] -> Prelookup/1
  Prelookup/2 -> AP_RollToYawRateLoop_Kp/4, AP_RollToYawRateLoop_Ki/4
  Prelookup/1 -> AP_RollToYawRateLoop_Kp/3, AP_RollToYawRateLoop_Ki/3
  [pres_alt_m] -> Prelookup3/1
  Prelookup3/2 -> AP_RollToYawRateLoop_Kp/2, AP_RollToYawRateLoop_Ki/2
  Prelookup3/1 -> AP_RollToYawRateLoop_Kp/1, AP_RollToYawRateLoop_Ki/1
  AP_RollToYawRateLoop_Kp/1 -> Product1/1
  AP_RollToYawRateLoop_Ki/1 -> Product2/1
  [DynPres_Pa] -> Prelookup2/1, Subsystem1/3(DynPres)
  [pres_alt_m] -> Prelookup1/1, Subsystem1/2(pres_alt_m)
  Prelookup1/1 -> AP_YawRateLoop_Ki/1, AP_YawRateLoop_Kp/1
  Prelookup1/2 -> AP_YawRateLoop_Ki/2, AP_YawRateLoop_Kp/2
  Prelookup2/1 -> AP_YawRateLoop_Ki/3, AP_YawRateLoop_Kp/3
  Prelookup2/2 -> AP_YawRateLoop_Ki/4, AP_YawRateLoop_Kp/4
  AP_YawRateLoop_ErrLPF/1 -> Product3/1, AP_YawRateLoop_Kd/1, Subsystem1/1(u)
  Subsystem1/1(y) -> Product4/1
  AP_YawRateLoop_Kp/1 -> Product4/2
  AP_YawRateLoop_Ki/1 -> Product3/2

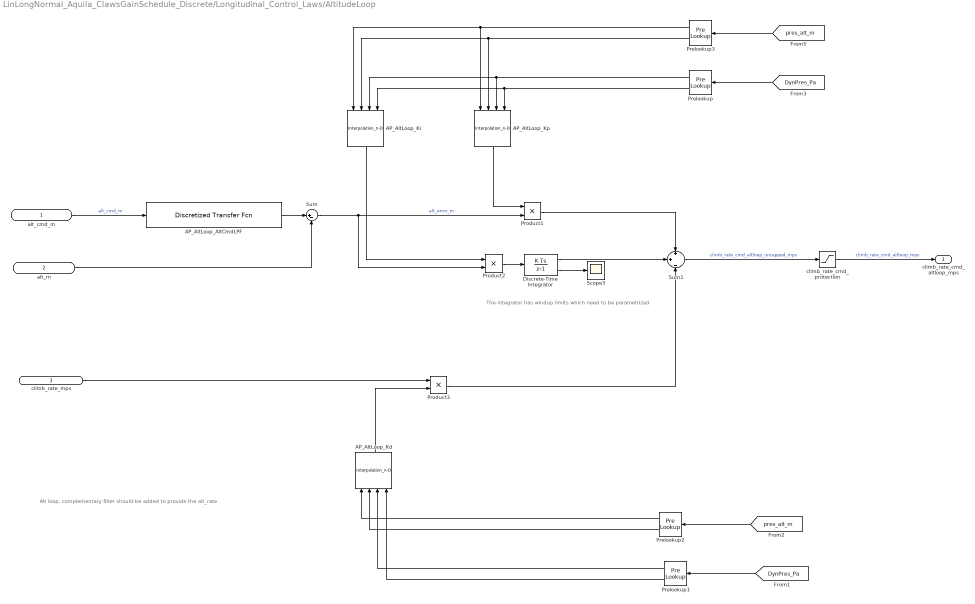
== system LinLongNormal_Aquila_ClawsGainSchedule_Discrete/Longitudinal_Control_Laws/AltitudeLoop ==
  note: The integrator has windup limits which need to be parametrized
  note: Alt loop,
      | complementary filter should be added to provide the alt_rate
  alt_cmd_m : Inport
  alt_m : Inport  Port=2
  climb_rate_mps : Inport  Port=3
  AP_AltLoop_AltCmdLPF : discretizing/Discretized Transfer Fcn  Numerator=[1]  Denominator=[AP_AltLoop_AltCmdLPFDenTau 1]  AbsTol=auto  SampleTime=Ts  method=zoh  Wc=1
  AP_AltLoop_Kd : Interpolation_n-D  Table=AP_AltLoop_Kd0  InternalRulePriority=Speed
  AP_AltLoop_Ki : Interpolation_n-D  Table=AP_AltLoop_Ki0  InternalRulePriority=Speed
  AP_AltLoop_Kp : Interpolation_n-D  Table=AP_AltLoop_Kp0  InternalRulePriority=Speed
  Discrete-Time Integrator : DiscreteIntegrator  InitialConditionSetting=State (most efficient)  SampleTime=-1  LimitOutput=on  UpperSaturationLimit=AP_AltLoop_Ki_WindupMaxLim  LowerSaturationLimit=AP_AltLoop_Ki_WindupMinLim  ShowSaturationPort=on  ICPrevOutput=DiscIntNeverNeededParam  ICPrevScaledInput=DiscIntNeverNeededParam
  Prelookup : PreLookup  BreakpointsData=45:15:150  ExtrapMethod=Linear
  Prelookup1 : PreLookup  BreakpointsData=45:15:150  ExtrapMethod=Linear
  Prelookup2 : PreLookup  BreakpointsData=0:1500:12000  ExtrapMethod=Linear
  Prelookup3 : PreLookup  BreakpointsData=0:1500:12000  ExtrapMethod=Linear
  Product1 : Product
  Product2 : Product
  Product3 : Product
  Scope3 : Scope
  Sum : Sum  Inputs=|+-
  Sum1 : Sum  Inputs=+|+|-
  climb_rate_cmd_protection : Saturate  UpperLimit=AP_TASLoop_MaxClimbRateCmdmps  LowerLimit=AP_TASLoop_MinClimbRateCmdmps
  climb_rate_cmd_altloop_mps : Outport
  wires:
  Product2/1 -> Discrete-Time Integrator/1
  Sum/1 -> Product1/2, Product2/2  "alt_error_m"
  Product1/1 -> Sum1/1
  Discrete-Time Integrator/1 -> Sum1/2
  alt_cmd_m/1 -> AP_AltLoop_AltCmdLPF/1  "alt_cmd_m"
  AP_AltLoop_AltCmdLPF/1 -> Sum/1
  alt_m/1 -> Sum/2
  Sum1/1 -> climb_rate_cmd_protection/1  "climb_rate_cmd_altloop_uncapped_mps"
  climb_rate_mps/1 -> Product3/1
  climb_rate_cmd_protection/1 -> climb_rate_cmd_altloop_mps/1  "climb_rate_cmd_altloop_mps"
  Discrete-Time Integrator/2 -> Scope3/1
  [DynPres_Pa] -> Prelookup/1
  Prelookup/2 -> AP_AltLoop_Ki/4, AP_AltLoop_Kp/4
  Prelookup/1 -> AP_AltLoop_Ki/3, AP_AltLoop_Kp/3
  [pres_alt_m] -> Prelookup3/1
  Prelookup3/1 -> AP_AltLoop_Ki/1, AP_AltLoop_Kp/1
  Prelookup3/2 -> AP_AltLoop_Ki/2, AP_AltLoop_Kp/2
  AP_AltLoop_Kp/1 -> Product1/1
  AP_AltLoop_Ki/1 -> Product2/1
  [DynPres_Pa] -> Prelookup1/1
  Prelookup1/2 -> AP_AltLoop_Kd/4
  Prelookup1/1 -> AP_AltLoop_Kd/3
  [pres_alt_m] -> Prelookup2/1
  Prelookup2/1 -> AP_AltLoop_Kd/1
  Prelookup2/2 -> AP_AltLoop_Kd/2
  AP_AltLoop_Kd/1 -> Product3/2
  Product3/1 -> Sum1/3

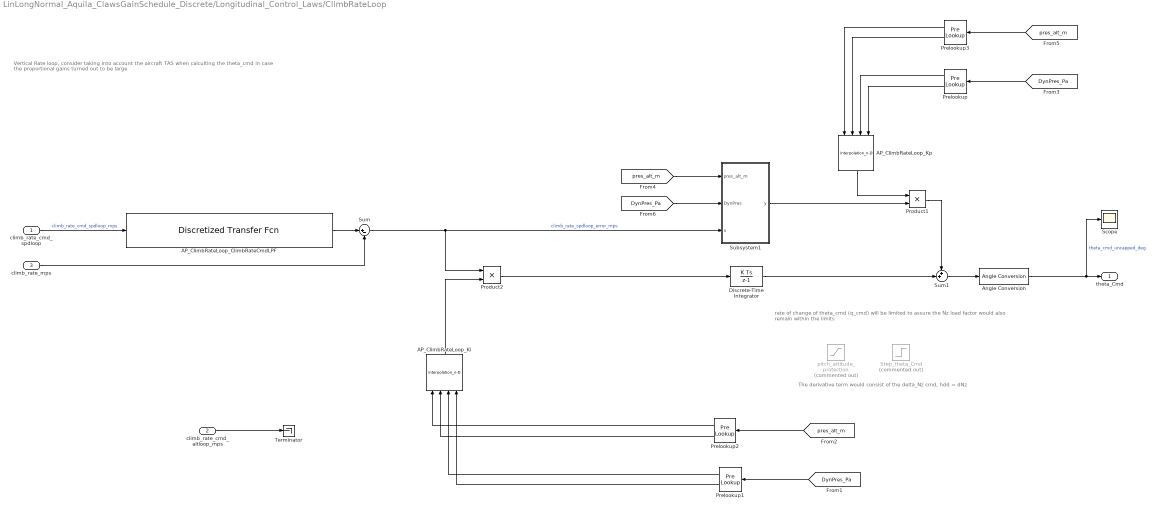
== system LinLongNormal_Aquila_ClawsGainSchedule_Discrete/Longitudinal_Control_Laws/ClimbRateLoop ==
  note: rate of change of theta_cmd (q_cmd) will be limited to
      | assure the Nz load factor would also remain within the limits
  note: Vertical Rate loop,
      | consider taking into account the aircraft TAS when calculting the theta_cmd in case the proportional gains turned out to be large
  note: The derivative term would consist of the delta_Nz cmd, hdd = dNz
  climb_rate_cmd_spdloop : Inport
  climb_rate_cmd_altloop_mps : Inport  Port=2
  climb_rate_mps : Inport  Port=3
  AP_ClimbRateLoop_ClimbRateCmdLPF : discretizing/Discretized Transfer Fcn  Numerator=[1]  Denominator=[AP_ClimbRateLoop_ClimbRateCmdLPFDenTau 1]  AbsTol=auto  SampleTime=0.04  method=zoh  Wc=1
  AP_ClimbRateLoop_Ki : Interpolation_n-D  Table=AP_ClimbRateLoop_Ki0  InternalRulePriority=Speed
  AP_ClimbRateLoop_Kp : Interpolation_n-D  Table=AP_ClimbRateLoop_Kp0  InternalRulePriority=Speed
  Angle Conversion : aerolibconvert2/Angle Conversion  IU=rad  OU=deg
  Discrete-Time Integrator : DiscreteIntegrator  InitialConditionSetting=State (most efficient)  SampleTime=-1  ICPrevOutput=DiscIntNeverNeededParam  ICPrevScaledInput=DiscIntNeverNeededParam
  Prelookup : PreLookup  BreakpointsData=45:15:150  ExtrapMethod=Linear
  Prelookup1 : PreLookup  BreakpointsData=45:15:150  ExtrapMethod=Linear
  Prelookup2 : PreLookup  BreakpointsData=0:1500:12000  ExtrapMethod=Linear
  Prelookup3 : PreLookup  BreakpointsData=0:1500:12000  ExtrapMethod=Linear
  Product1 : Product
  Product2 : Product
  Scope : Scope
  Step_theta_Cmd : Step  Commented=on  SampleTime=0
  Subsystem1 : Subsystem
  Sum : Sum  Inputs=|+-
  Sum1 : Sum  Inputs=++|
  Terminator : Terminator
  pitch_attitude_protection : Saturate  Commented=on  UpperLimit=AP_ClimbRateLoop_MaxPitchCmdrad  LowerLimit=AP_ClimbRateLoop_MinPitchCmdrad
  theta_Cmd : Outport
  wires:
  climb_rate_mps/1 -> Sum/2
  Sum1/1 -> Angle Conversion/1
  Product2/1 -> Discrete-Time Integrator/1
  Sum/1 -> Subsystem1/3(u), Product2/1  "climb_rate_spdloop_error_mps"
  Product1/1 -> Sum1/1
  Discrete-Time Integrator/1 -> Sum1/2
  climb_rate_cmd_spdloop/1 -> AP_ClimbRateLoop_ClimbRateCmdLPF/1  "climb_rate_cmd_spdloop_mps"
  Angle Conversion/1 -> theta_Cmd/1, Scope/1  "theta_cmd_uncapped_deg"
  AP_ClimbRateLoop_ClimbRateCmdLPF/1 -> Sum/1
  [DynPres_Pa] -> Prelookup/1
  Prelookup/2 -> AP_ClimbRateLoop_Kp/4
  Prelookup/1 -> AP_ClimbRateLoop_Kp/3
  [pres_alt_m] -> Prelookup3/1
  Prelookup3/1 -> AP_ClimbRateLoop_Kp/1
  Prelookup3/2 -> AP_ClimbRateLoop_Kp/2
  AP_ClimbRateLoop_Kp/1 -> Product1/1
  climb_rate_cmd_altloop_mps/1 -> Terminator/1
  [DynPres_Pa] -> Prelookup1/1
  Prelookup1/2 -> AP_ClimbRateLoop_Ki/4
  Prelookup1/1 -> AP_ClimbRateLoop_Ki/3
  [pres_alt_m] -> Prelookup2/1
  Prelookup2/1 -> AP_ClimbRateLoop_Ki/1
  Prelookup2/2 -> AP_ClimbRateLoop_Ki/2
  AP_ClimbRateLoop_Ki/1 -> Product2/2
  [pres_alt_m] -> Subsystem1/1(pres_alt_m)
  [DynPres_Pa] -> Subsystem1/2(DynPres)
  Subsystem1/1(y) -> Product1/2

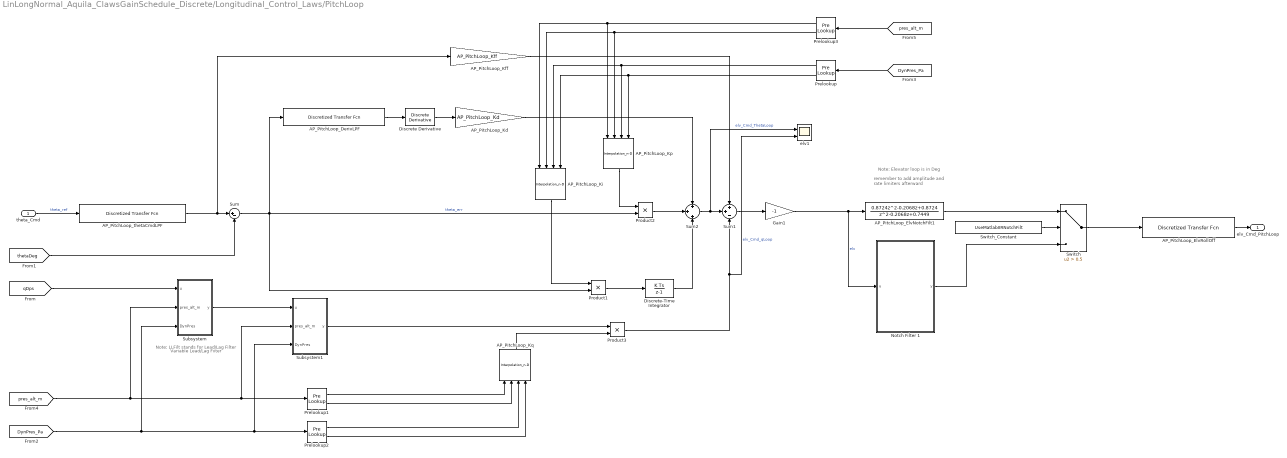
== system LinLongNormal_Aquila_ClawsGainSchedule_Discrete/Longitudinal_Control_Laws/PitchLoop ==
  note: Variable Lead/Lag Filter
  note: remember to add amplitude and
      | rate limiters afterward
  note: Note: Elevator loop is in Deg
  note: Note: LLFilt stands for Lead/Lag Filter
  theta_Cmd : Inport
  AP_PitchLoop_DerivLPF : discretizing/Discretized Transfer Fcn  Numerator=[1]  Denominator=[AP_PitchLoop_DerivLPFDenTau 1]  AbsTol=auto  SampleTime=0.04  method=zoh  Wc=1
  AP_PitchLoop_ElvNotchFilt1 : DiscreteTransferFcn  Numerator=[0.8724 -0.2068 0.8724]  Denominator=[1 -0.2068 0.7449]  SampleTime=Ts
  AP_PitchLoop_ElvRollOff : discretizing/Discretized Transfer Fcn  Numerator=[AP_PitchLoop_wn_ElvRollOff^2]  Denominator=[1 2*AP_PitchLoop_zeta_ElvRollOff*AP_PitchLoop_wn_ElvRollOff AP_PitchLoop_wn_ElvRollOff^2]  AbsTol=auto  SampleTime=0.04  method=zoh  Wc=1
  AP_PitchLoop_Kd : Gain  Gain=AP_PitchLoop_Kd
  AP_PitchLoop_Kff : Gain  Gain=AP_PitchLoop_Kff
  AP_PitchLoop_Ki : Interpolation_n-D  Table=AP_PitchLoop_Ki0  InternalRulePriority=Speed
  AP_PitchLoop_Kp : Interpolation_n-D  Table=AP_PitchLoop_Kp0  InternalRulePriority=Speed
  AP_PitchLoop_Kq : Interpolation_n-D  Table=AP_PitchLoop_Kq0  InternalRulePriority=Speed
  AP_PitchLoop_thetaCmdLPF : discretizing/Discretized Transfer Fcn  Numerator=[1]  Denominator=[AP_PitchLoop_thetaCmdLPFDenTau 1]  AbsTol=auto  SampleTime=0.04  method=zoh  Wc=1
  Discrete Derivative : simulink/Discrete/Discrete Derivative  gainval=1.0  ICPrevScaledInput=0.0  OutMin=[]  OutMax=[]  OutDataType=fixdt(1, 16)  OutScaling=2^-10  DoSatur=off
  Discrete-Time Integrator : DiscreteIntegrator  InitialConditionSetting=State (most efficient)  SampleTime=-1  ICPrevOutput=DiscIntNeverNeededParam  ICPrevScaledInput=DiscIntNeverNeededParam
  Gain1 : Gain  Gain=-1
  Notch Filter 1 : Subsystem
  Prelookup : PreLookup  BreakpointsData=45:15:150  ExtrapMethod=Linear
  Prelookup1 : PreLookup  BreakpointsData=0:1500:12000  ExtrapMethod=Linear
  Prelookup2 : PreLookup  BreakpointsData=45:15:150  ExtrapMethod=Linear
  Prelookup3 : PreLookup  BreakpointsData=0:1500:12000  ExtrapMethod=Linear
  Product1 : Product
  Product2 : Product
  Product3 : Product
  Subsystem : Subsystem
  Subsystem1 : Subsystem
  Sum : Sum  Inputs=|+-
  Sum1 : Sum  Inputs=++-
  Sum2 : Sum  Inputs=+|+|+
  Switch : Switch  Criteria=u2 > Threshold  Threshold=0.5
  Switch_Constant : Constant  Value=UseMatlabIIRNotchFilt
  elv1 : Scope  NumInputPorts=2
  elv_Cmd_PitchLoop : Outport
  wires:
  Sum/1 -> Product2/2, AP_PitchLoop_DerivLPF/1, Product1/2  "theta_err"
  Product1/1 -> Discrete-Time Integrator/1
  Product3/1 -> elv1/2, Sum1/3  "elv_Cmd_qLoop"
  AP_PitchLoop_Kff/1 -> Sum1/1
  [thetaDeg] -> Sum/2
  Sum2/1 -> Sum1/2, elv1/1  "elv_Cmd_ThetaLoop"
  Sum1/1 -> Gain1/1
  theta_Cmd/1 -> AP_PitchLoop_thetaCmdLPF/1  "theta_ref"
  AP_PitchLoop_ElvRollOff/1 -> elv_Cmd_PitchLoop/1
  Discrete Derivative/1 -> AP_PitchLoop_Kd/1
  AP_PitchLoop_DerivLPF/1 -> Discrete Derivative/1
  Discrete-Time Integrator/1 -> Sum2/3
  AP_PitchLoop_Kd/1 -> Sum2/1
  Switch/1 -> AP_PitchLoop_ElvRollOff/1
  AP_PitchLoop_thetaCmdLPF/1 -> Sum/1, AP_PitchLoop_Kff/1
  AP_PitchLoop_Kp/1 -> Product2/1
  Product2/1 -> Sum2/2
  [DynPres_Pa] -> Prelookup/1
  AP_PitchLoop_Ki/1 -> Product1/1
  [DynPres_Pa] -> Prelookup2/1, Subsystem1/3(DynPres), Subsystem/3(DynPres)
  AP_PitchLoop_Kq/1 -> Product3/2
  [qDps] -> Subsystem/1(u)
  [pres_alt_m] -> Prelookup1/1, Subsystem1/2(pres_alt_m), Subsystem/2(pres_alt_m)
  Prelookup1/1 -> AP_PitchLoop_Kq/1
  Prelookup1/2 -> AP_PitchLoop_Kq/2
  Prelookup2/1 -> AP_PitchLoop_Kq/3
  Prelookup2/2 -> AP_PitchLoop_Kq/4
  Prelookup/2 -> AP_PitchLoop_Kp/4, AP_PitchLoop_Ki/4
  Prelookup/1 -> AP_PitchLoop_Kp/3, AP_PitchLoop_Ki/3
  [pres_alt_m] -> Prelookup3/1
  Prelookup3/1 -> AP_PitchLoop_Ki/1, AP_PitchLoop_Kp/1
  Prelookup3/2 -> AP_PitchLoop_Kp/2, AP_PitchLoop_Ki/2
  Subsystem1/1(y) -> Product3/1
  Subsystem/1(y) -> Subsystem1/1(u)
  AP_PitchLoop_ElvNotchFilt1/1 -> Switch/1
  Gain1/1 -> AP_PitchLoop_ElvNotchFilt1/1, Notch Filter 1/1(u)  "elv"
  Notch Filter 1/1(y) -> Switch/3
  Switch_Constant/1 -> Switch/2

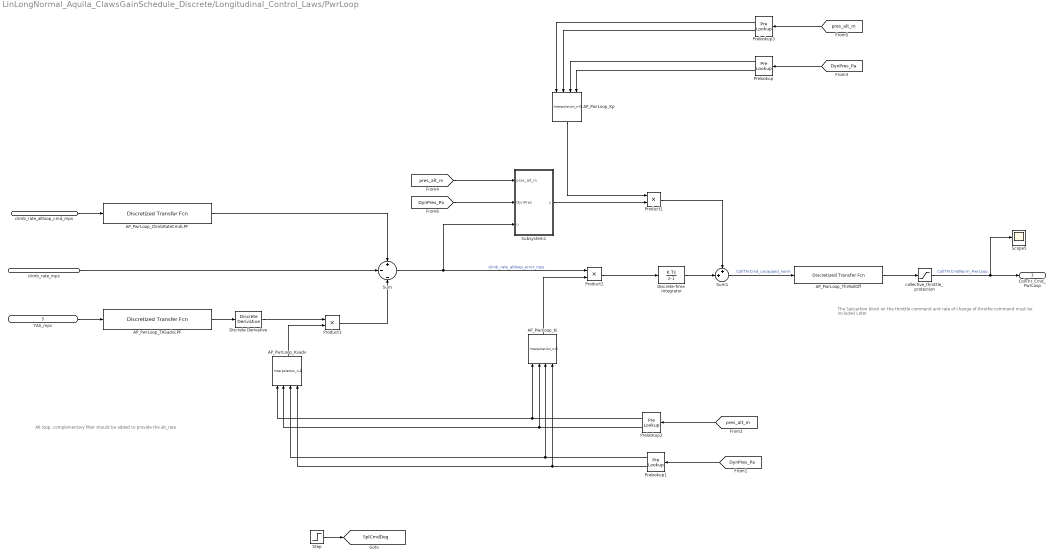
== system LinLongNormal_Aquila_ClawsGainSchedule_Discrete/Longitudinal_Control_Laws/PwrLoop ==
  note: The Satuartion block on the throttle command and rate of change of throttle command must be
      | included Later
  note: Alt loop,
      | complementary filter should be added to provide the alt_rate
  climb_rate_altloop_cmd_mps : Inport
  climb_rate_mps : Inport  Port=2
  TAS_mps : Inport  Port=3
  AP_PwrLoop_ClimbRateCmdLPF : discretizing/Discretized Transfer Fcn  Numerator=[1]  Denominator=[AP_PwrLoop_ClimbRateCmdLPFDenTau 1]  AbsTol=auto  SampleTime=Ts  method=zoh  Wc=1
  AP_PwrLoop_Ki : Interpolation_n-D  Table=AP_PwrLoop_Ki0  InternalRulePriority=Speed
  AP_PwrLoop_Kp : Interpolation_n-D  Table=AP_PwrLoop_Kp0  InternalRulePriority=Speed
  AP_PwrLoop_Kvadv : Interpolation_n-D  Table=AP_PwrLoop_Kvadv0  InternalRulePriority=Speed
  AP_PwrLoop_TASadvLPF : discretizing/Discretized Transfer Fcn  Numerator=[1]  Denominator=[AP_TASLoop_TASadvLPFDenTau 1]  AbsTol=auto  SampleTime=Ts  method=zoh  Wc=1
  AP_PwrLoop_ThrRollOff : discretizing/Discretized Transfer Fcn  Numerator=[AP_PwrLoop_wn_ThrRollOff^2]  Denominator=[1 2*AP_PwrLoop_zeta_ThrRollOff*AP_PwrLoop_wn_ThrRollOff AP_PwrLoop_wn_ThrRollOff^2]  AbsTol=auto  SampleTime=0.04  method=zoh  Wc=1
  Discrete Derivative : simulink/Discrete/Discrete Derivative  gainval=1.0  ICPrevScaledInput=0.0  OutMin=[]  OutMax=[]  OutDataType=fixdt(1, 16)  OutScaling=2^-10  DoSatur=off
  Discrete-Time Integrator : DiscreteIntegrator  InitialConditionSetting=State (most efficient)  SampleTime=-1  ICPrevOutput=DiscIntNeverNeededParam  ICPrevScaledInput=DiscIntNeverNeededParam
  Prelookup : PreLookup  BreakpointsData=45:15:150  ExtrapMethod=Linear
  Prelookup1 : PreLookup  BreakpointsData=45:15:150  ExtrapMethod=Linear
  Prelookup2 : PreLookup  BreakpointsData=0:1500:12000  ExtrapMethod=Linear
  Prelookup3 : PreLookup  BreakpointsData=0:1500:12000  ExtrapMethod=Linear
  Product1 : Product
  Product2 : Product
  Product3 : Product
  Scope5 : Scope
  Step : Step  After=0  SampleTime=0
  Subsystem1 : Subsystem
  Sum : Sum  Inputs=+|-|-
  Sum1 : Sum  Inputs=++|
  collective_throttle_protection : Saturate  UpperLimit=AP_PwrLoop_MaxThrCmdNorm  LowerLimit=AP_PwrLoop_MinThrCmdNorm
  CollThr_Cmd_PwrLoop : Outport
  tag scope: SplCmdDeg=global
  wires:
  Product2/1 -> Discrete-Time Integrator/1
  Sum/1 -> Product2/1, Subsystem1/3(u)  "climb_rate_altloop_error_mps"
  Product1/1 -> Sum1/1
  Discrete-Time Integrator/1 -> Sum1/2
  climb_rate_altloop_cmd_mps/1 -> AP_PwrLoop_ClimbRateCmdLPF/1
  AP_PwrLoop_ClimbRateCmdLPF/1 -> Sum/1
  climb_rate_mps/1 -> Sum/2
  Sum1/1 -> AP_PwrLoop_ThrRollOff/1  "CollThrCmd_uncapped_norm"
  AP_PwrLoop_TASadvLPF/1 -> Discrete Derivative/1
  Discrete Derivative/1 -> Product3/1
  TAS_mps/1 -> AP_PwrLoop_TASadvLPF/1
  Product3/1 -> Sum/3
  collective_throttle_protection/1 -> Scope5/1, CollThr_Cmd_PwrLoop/1  "CollThrCmdNorm_PwrLoop"
  AP_PwrLoop_ThrRollOff/1 -> collective_throttle_protection/1
  [DynPres_Pa] -> Prelookup/1
  Prelookup/2 -> AP_PwrLoop_Kp/4
  Prelookup/1 -> AP_PwrLoop_Kp/3
  [pres_alt_m] -> Prelookup3/1
  Prelookup3/1 -> AP_PwrLoop_Kp/1
  Prelookup3/2 -> AP_PwrLoop_Kp/2
  AP_PwrLoop_Kp/1 -> Product1/1
  [pres_alt_m] -> Subsystem1/1(pres_alt_m)
  [DynPres_Pa] -> Subsystem1/2(DynPres)
  Subsystem1/1(y) -> Product1/2
  [DynPres_Pa] -> Prelookup1/1
  Prelookup1/2 -> AP_PwrLoop_Kvadv/4, AP_PwrLoop_Ki/4
  Prelookup1/1 -> AP_PwrLoop_Kvadv/3, AP_PwrLoop_Ki/3
  [pres_alt_m] -> Prelookup2/1
  Prelookup2/1 -> AP_PwrLoop_Kvadv/1, AP_PwrLoop_Ki/1
  Prelookup2/2 -> AP_PwrLoop_Kvadv/2, AP_PwrLoop_Ki/2
  AP_PwrLoop_Ki/1 -> Product2/2
  AP_PwrLoop_Kvadv/1 -> Product3/2
  Step/1 -> [SplCmdDeg]

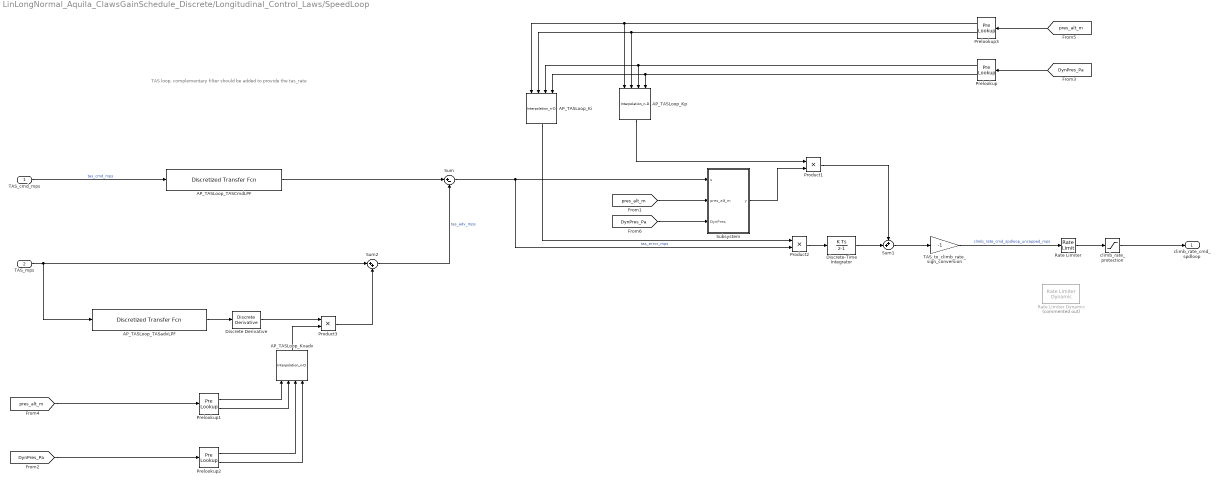
== system LinLongNormal_Aquila_ClawsGainSchedule_Discrete/Longitudinal_Control_Laws/SpeedLoop ==
  note: TAS loop,
      | complementary filter should be added to provide the tas_rate
  TAS_cmd_mps : Inport
  TAS_mps : Inport  Port=2
  AP_TASLoop_Ki : Interpolation_n-D  Table=AP_TASLoop_Ki0  InternalRulePriority=Speed
  AP_TASLoop_Kp : Interpolation_n-D  Table=AP_TASLoop_Kp0  InternalRulePriority=Speed
  AP_TASLoop_Kvadv : Interpolation_n-D  Table=AP_TASLoop_Kvadv0  InternalRulePriority=Speed
  AP_TASLoop_TASCmdLPF : discretizing/Discretized Transfer Fcn  Numerator=[1]  Denominator=[AP_TASLoop_TASCmdLPFDenTau 1]  AbsTol=auto  SampleTime=Ts  method=zoh  Wc=1
  AP_TASLoop_TASadvLPF : discretizing/Discretized Transfer Fcn  Numerator=[1]  Denominator=[AP_TASLoop_TASadvLPFDenTau 1]  AbsTol=auto  SampleTime=Ts  method=zoh  Wc=1
  Discrete Derivative : simulink/Discrete/Discrete Derivative  gainval=1.0  ICPrevScaledInput=0.0  OutMin=[]  OutMax=[]  OutDataType=fixdt(1, 16)  OutScaling=2^-10  DoSatur=off
  Discrete-Time Integrator : DiscreteIntegrator  InitialConditionSetting=State (most efficient)  SampleTime=-1  ICPrevOutput=DiscIntNeverNeededParam  ICPrevScaledInput=DiscIntNeverNeededParam
  Prelookup : PreLookup  BreakpointsData=45:15:150  ExtrapMethod=Linear
  Prelookup1 : PreLookup  BreakpointsData=0:1500:12000  ExtrapMethod=Linear
  Prelookup2 : PreLookup  BreakpointsData=45:15:150  ExtrapMethod=Linear
  Prelookup3 : PreLookup  BreakpointsData=0:1500:12000  ExtrapMethod=Linear
  Product1 : Product
  Product2 : Product
  Product3 : Product
  Rate Limiter : RateLimiter  RisingSlewLimit=AP_TASLoop_ClimbRateCmdRateLimMax  FallingSlewLimit=AP_TASLoop_ClimbRateCmdRateLimMin  SampleTimeMode=inherited
  Rate Limiter Dynamic : simulink/Discontinuities/Rate Limiter Dynamic  Commented=on
      settings: SourceProductName=Simulink
  Subsystem : Subsystem
  Sum : Sum  Inputs=|+-
  Sum1 : Sum  Inputs=++|
  Sum2 : Sum  Inputs=|++
  TAS_to_climb_rate_sign_conversion : Gain  Gain=-1
  climb_rate_protection : Saturate  UpperLimit=AP_TASLoop_MaxClimbRateCmdmps  LowerLimit=AP_TASLoop_MinClimbRateCmdmps
  climb_rate_cmd_spdloop : Outport
  wires:
  Product2/1 -> Discrete-Time Integrator/1
  Sum/1 -> Product2/2, Subsystem/1(u)  "tas_error_mps"
  Product1/1 -> Sum1/1
  Discrete-Time Integrator/1 -> Sum1/2
  TAS_cmd_mps/1 -> AP_TASLoop_TASCmdLPF/1  "tas_cmd_mps"
  TAS_mps/1 -> Sum2/1, AP_TASLoop_TASadvLPF/1
  AP_TASLoop_TASCmdLPF/1 -> Sum/1
  Sum2/1 -> Sum/2  "tas_adv_mps"
  AP_TASLoop_TASadvLPF/1 -> Discrete Derivative/1
  Discrete Derivative/1 -> Product3/1
  Product3/1 -> Sum2/2
  [DynPres_Pa] -> Prelookup/1
  Prelookup/2 -> AP_TASLoop_Ki/4, AP_TASLoop_Kp/4
  Prelookup/1 -> AP_TASLoop_Ki/3, AP_TASLoop_Kp/3
  [pres_alt_m] -> Prelookup3/1
  Prelookup3/1 -> AP_TASLoop_Ki/1, AP_TASLoop_Kp/1
  Prelookup3/2 -> AP_TASLoop_Ki/2, AP_TASLoop_Kp/2
  AP_TASLoop_Kp/1 -> Product1/1
  AP_TASLoop_Ki/1 -> Product2/1
  [DynPres_Pa] -> Prelookup2/1
  [pres_alt_m] -> Prelookup1/1
  Prelookup1/1 -> AP_TASLoop_Kvadv/1
  Prelookup1/2 -> AP_TASLoop_Kvadv/2
  Prelookup2/1 -> AP_TASLoop_Kvadv/3
  Prelookup2/2 -> AP_TASLoop_Kvadv/4
  AP_TASLoop_Kvadv/1 -> Product3/2
  [pres_alt_m] -> Subsystem/2(pres_alt_m)
  [DynPres_Pa] -> Subsystem/3(DynPres)
  Subsystem/1(y) -> Product1/2
  Sum1/1 -> TAS_to_climb_rate_sign_conversion/1
  TAS_to_climb_rate_sign_conversion/1 -> Rate Limiter/1  "climb_rate_cmd_spdloop_uncapped_mps"
  climb_rate_protection/1 -> climb_rate_cmd_spdloop/1
  Rate Limiter/1 -> climb_rate_protection/1

== system LinLongNormal_Aquila_ClawsGainSchedule_Discrete/Lateral_Directional_Control_Laws/GndTrkLoop/pi Bound ==
  In : Inport
  2pi : Constant  Value=2*pi
  Math Function : Math  Operator=mod  SaturateOnIntegerOverflow=on
  Sum1 : Sum  Inputs=|+-  SaturateOnIntegerOverflow=on  InputSameDT=on  OutDataTypeStr=Inherit: Same as first input
  Sum2 : Sum  Inputs=|++  SaturateOnIntegerOverflow=on  InputSameDT=on  OutDataTypeStr=Inherit: Same as first input
  pi : Constant  Value=pi
  Out : Outport
  wires:
  Sum1/1 -> Out/1
  pi/1 -> Sum1/2, Sum2/2
  Sum2/1 -> Math Function/1
  In/1 -> Sum2/1
  2pi/1 -> Math Function/2
  Math Function/1 -> Sum1/1
